simulink model "Sistema_Teste_Hugo_1"  (R2019a)
settings: Solver=ode23t  StartTime=0.0  StopTime=86400  MaxStep=6  RelTol=1e-3  EnableMultiTasking=on
InitFcn:
  | Dados_do_Sistema
undefined symbols (not defined in the file or in its folder): D1, Dados, Delta
libraries: powerlib x263, powerlib_meascontrol x79, dspsrcs4 x50
(part 5 of 5)

== system Sistema_Teste_Hugo_1/Load_8 ==
  note: Subsystem
  Add{,1..5} (6 alike) : Sum
  Ativa : Sin  Amplitude=16  Frequency=6.9e-5  Phase=-3.14  SampleTime=0
  Complex to Magnitude-Angle : ComplexToMagnitudeAngle  Output=Angle
  Constant2 : Constant  Value=-1.57079
  Controlled Current Source : powerlib/Electrical Sources/Controlled Current Source  Initialize=off  Source_Type=AC  Amplitude=0  Phase=0  Frequency=0  Measurements=None
      settings: SourceProductName=Simscape Electrical
  Controlled Current Source1 : powerlib/Electrical Sources/Controlled Current Source  Initialize=off  Source_Type=AC  Amplitude=0  Phase=0  Frequency=0  Measurements=None
      settings: SourceProductName=Simscape Electrical
  Controlled Current Source2 : powerlib/Electrical Sources/Controlled Current Source  Initialize=off  Source_Type=AC  Amplitude=0  Phase=0  Frequency=0  Measurements=None
      settings: SourceProductName=Simscape Electrical
  Demux : Demux  Outputs=3
  Demux1 : Demux  Outputs=3
  Demux2 : Demux  Outputs=3
  First-Order Filter : powerlib_meascontrol/Filters/First-Order Filter  FilterType=Lowpass  Tc=200  Ts=0  Initialize=on  Vac_Init=[0, 0, 60]  Vdc_Init=1  PlotResponse=off  FreqRange="[0,  200,  1]"
      settings: SourceProductName=Simscape Electrical
  First-Order Filter1 : powerlib_meascontrol/Filters/First-Order Filter  FilterType=Lowpass  Tc=400  Ts=0  Initialize=on  Vac_Init=[0, 0, 60]  Vdc_Init=1  PlotResponse=off  FreqRange="[0,  200,  1]"
      settings: SourceProductName=Simscape Electrical
  Gain : Gain  Gain=0.25
  Gain1 : Gain  Gain=0.25
  Gain4 : Gain  Gain=-1
  Ground2 : powerlib/Elements/Ground  LConnTagsString=a
      settings: SourceProductName=Simscape Electrical
  Magnitude-Angle to Complex{,1..5} (6 alike) : MagnitudeAngleToComplex
  Memory1 : Memory
  Memory2 : Memory
  Mux1 : Mux  Inputs=3
  Power (Phasor)2 : powerlib_meascontrol/Measurements/Power (Phasor)
      settings: SourceProductName=Simscape Electrical  SourceProductBaseCode=PS
  Product : Product
  Product1 : Product
  Random Source : dspsrcs4/Random Source  SrcType=Uniform  NormMethod=Ziggurat  CltLength=12  MinVal=0.45  MaxVal=1  MeanVal=0  VarVal=1  RepMode=Repeatable  rawSeed=1  IsInherit=off  SampMode=Discrete  SampTime=200  SampFrame=1  DataType=Single  OutComplex=Real  OutputFrames=on
  Random Source1 : dspsrcs4/Random Source  SrcType=Uniform  NormMethod=Ziggurat  CltLength=12  MinVal=0.75  MaxVal=1  MeanVal=0  VarVal=1  RepMode=Repeatable  rawSeed=1  IsInherit=off  SampMode=Discrete  SampTime=400  SampFrame=1  DataType=Single  OutComplex=Real  OutputFrames=on
  Reativa : Sin  Amplitude=5  Frequency=6.9e-5  Phase=-3.14  SampleTime=0
  Saturation : Saturate  UpperLimit=36  LowerLimit=7
  Saturation1 : Saturate  UpperLimit=10  LowerLimit=3.5
  Three-Phase Series RLC Branch2 : powerlib/Elements/Three-Phase Series RLC Branch  LConnTagsString=A|B|C  RConnTagsString=A|B|C  BranchType=RC  Resistance=0.0001  Inductance=5.46e-6  Capacitance=1e-9  Measurements=None
      settings: SourceProductName=Simscape Electrical
  Three-Phase V-I Measurement2 : powerlib/Measurements/Three-Phase V-I Measurement  VoltageMeasurement=phase-to-ground  SetLabelV=on  LabelV=VL8  Vpu=off  VpuLL=off  CurrentMeasurement=no  SetLabelI=on  LabelI=IL8  Ipu=off  Pbase=100e6  Vbase=500e3  OutputType=Complex  PhasorSimulation=on  PSBequivalent=0
      settings: SourceProductName=Simscape Electrical
  To Workspace1 : ToWorkspace  VariableName=P_Load_8_A  SampleTime=-1
  To Workspace2 : ToWorkspace  VariableName=Q_Load_8_A  SampleTime=-1
  To Workspace3 : ToWorkspace  VariableName=P_Load_8_B  SampleTime=-1
  To Workspace4 : ToWorkspace  VariableName=P_Load_8_C  SampleTime=-1
  To Workspace5 : ToWorkspace  VariableName=Q_Load_8_B  SampleTime=-1
  To Workspace6 : ToWorkspace  VariableName=Q_Load_8_C  SampleTime=-1
  i_current1 : powerlib/Measurements/Current Measurement  PhasorSimulation=on  OutputType=Complex  PSBequivalent=0
      settings: SourceProductName=Simscape Electrical
  i_current2 : powerlib/Measurements/Current Measurement  PhasorSimulation=on  OutputType=Complex  PSBequivalent=0
      settings: SourceProductName=Simscape Electrical
  i_current3 : powerlib/Measurements/Current Measurement  PhasorSimulation=on  OutputType=Complex  PSBequivalent=0
      settings: SourceProductName=Simscape Electrical
  a+ : PMIOPort  Side=Right
  b+ : PMIOPort  Port=2  Side=Right
  c+ : PMIOPort  Port=3  Side=Right
  wires:
  Ativa/1 -> Saturation/1
  Saturation/1 -> Product/2
  Random Source/1 -> First-Order Filter/1
  First-Order Filter/1 -> Product/1
  Reativa/1 -> Saturation1/1
  First-Order Filter1/1 -> Product1/1
  Random Source1/1 -> First-Order Filter1/1
  Saturation1/1 -> Product1/2
  Add/1 -> Controlled Current Source/1
  Magnitude-Angle to Complex/1 -> Add/1
  Magnitude-Angle to Complex1/1 -> Add/2
  Add1/1 -> Controlled Current Source1/1
  Magnitude-Angle to Complex2/1 -> Add1/1
  Magnitude-Angle to Complex3/1 -> Add1/2
  Add2/1 -> Controlled Current Source2/1
  Magnitude-Angle to Complex4/1 -> Add2/1
  Magnitude-Angle to Complex5/1 -> Add2/2
  Complex to Magnitude-Angle/1 -> Demux/1
  Demux/1 -> Magnitude-Angle to Complex/2, Add3/2
  Constant2/1 -> Add5/1, Add4/1, Add3/1
  Add3/1 -> Magnitude-Angle to Complex1/2
  Demux/2 -> Add4/2, Magnitude-Angle to Complex2/2
  Add4/1 -> Magnitude-Angle to Complex3/2
  Demux/3 -> Magnitude-Angle to Complex4/2, Add5/2
  Add5/1 -> Magnitude-Angle to Complex5/2
  [VL8] -> Gain4/1
  Memory1/1 -> Complex to Magnitude-Angle/1
  Product/1 -> Gain1/1, Magnitude-Angle to Complex4/1, Magnitude-Angle to Complex2/1
  Product1/1 -> Gain/1, Magnitude-Angle to Complex5/1, Magnitude-Angle to Complex3/1
  Gain1/1 -> Magnitude-Angle to Complex/1
  Gain/1 -> Magnitude-Angle to Complex1/1
  Gain4/1 -> Memory1/1
  Mux1/1 -> Power (Phasor)2/2
  Power (Phasor)2/2 -> Demux2/1
  [VL8] -> Memory2/1
  i_current1/1 -> Mux1/2
  Power (Phasor)2/1 -> Demux1/1
  Demux2/1 -> To Workspace2/1
  Demux1/2 -> To Workspace3/1
  i_current2/1 -> Mux1/3
  Demux2/3 -> To Workspace6/1
  Demux2/2 -> To Workspace5/1
  Demux1/3 -> To Workspace4/1
  Memory2/1 -> Power (Phasor)2/1
  Demux1/1 -> To Workspace1/1
  i_current3/1 -> Mux1/1
  connections:
  Three-Phase V-I Measurement2/RConn1 -- Controlled Current Source/RConn1 -- Three-Phase Series RLC Branch2/LConn1
  Three-Phase V-I Measurement2/RConn2 -- Controlled Current Source1/RConn1 -- Three-Phase Series RLC Branch2/LConn2
  Three-Phase V-I Measurement2/RConn3 -- Controlled Current Source2/RConn1 -- Three-Phase Series RLC Branch2/LConn3
  Controlled Current Source1/LConn1 -- Three-Phase Series RLC Branch2/RConn3 -- Three-Phase Series RLC Branch2/RConn1 -- Controlled Current Source/LConn1 -- Three-Phase Series RLC Branch2/RConn2 -- Ground2/LConn1 -- Controlled Current Source2/LConn1
  a+/RConn1 -- i_current3/RConn1
  Three-Phase V-I Measurement2/LConn3 -- i_current2/LConn1
  b+/RConn1 -- i_current1/RConn1
  Three-Phase V-I Measurement2/LConn1 -- i_current3/LConn1
  c+/RConn1 -- i_current2/RConn1
  Three-Phase V-I Measurement2/LConn2 -- i_current1/LConn1

== system Sistema_Teste_Hugo_1/Load_9 ==
  note: Subsystem
  Add{,1..5} (6 alike) : Sum
  Ativa : Sin  Amplitude=8  Frequency=6.9e-5  Phase=-3.14  SampleTime=0
  Complex to Magnitude-Angle : ComplexToMagnitudeAngle  Output=Angle
  Constant2 : Constant  Value=-1.57079
  Controlled Current Source : powerlib/Electrical Sources/Controlled Current Source  Initialize=off  Source_Type=AC  Amplitude=0  Phase=0  Frequency=0  Measurements=None
      settings: SourceProductName=Simscape Electrical
  Controlled Current Source1 : powerlib/Electrical Sources/Controlled Current Source  Initialize=off  Source_Type=AC  Amplitude=0  Phase=0  Frequency=0  Measurements=None
      settings: SourceProductName=Simscape Electrical
  Controlled Current Source2 : powerlib/Electrical Sources/Controlled Current Source  Initialize=off  Source_Type=AC  Amplitude=0  Phase=0  Frequency=0  Measurements=None
      settings: SourceProductName=Simscape Electrical
  Demux : Demux  Outputs=3
  Demux1 : Demux  Outputs=3
  Demux2 : Demux  Outputs=3
  First-Order Filter : powerlib_meascontrol/Filters/First-Order Filter  FilterType=Lowpass  Tc=200  Ts=0  Initialize=on  Vac_Init=[0, 0, 60]  Vdc_Init=1  PlotResponse=off  FreqRange="[0,  200,  1]"
      settings: SourceProductName=Simscape Electrical
  First-Order Filter1 : powerlib_meascontrol/Filters/First-Order Filter  FilterType=Lowpass  Tc=400  Ts=0  Initialize=on  Vac_Init=[0, 0, 60]  Vdc_Init=1  PlotResponse=off  FreqRange="[0,  200,  1]"
      settings: SourceProductName=Simscape Electrical
  Gain : Gain  Gain=0.5
  Gain1 : Gain  Gain=0.5
  Gain4 : Gain  Gain=-1
  Ground2 : powerlib/Elements/Ground  LConnTagsString=a
      settings: SourceProductName=Simscape Electrical
  Magnitude-Angle to Complex{,1..5} (6 alike) : MagnitudeAngleToComplex
  Memory1 : Memory
  Memory2 : Memory
  Mux1 : Mux  Inputs=3
  Power (Phasor)2 : powerlib_meascontrol/Measurements/Power (Phasor)
      settings: SourceProductName=Simscape Electrical  SourceProductBaseCode=PS
  Product : Product
  Product1 : Product
  Random Source : dspsrcs4/Random Source  SrcType=Uniform  NormMethod=Ziggurat  CltLength=12  MinVal=0.8  MaxVal=1  MeanVal=0  VarVal=1  RepMode=Repeatable  rawSeed=1  IsInherit=off  SampMode=Discrete  SampTime=200  SampFrame=1  DataType=Single  OutComplex=Real  OutputFrames=on
  Random Source1 : dspsrcs4/Random Source  SrcType=Uniform  NormMethod=Ziggurat  CltLength=12  MinVal=0.5  MaxVal=1  MeanVal=0  VarVal=1  RepMode=Repeatable  rawSeed=1  IsInherit=off  SampMode=Discrete  SampTime=400  SampFrame=1  DataType=Single  OutComplex=Real  OutputFrames=on
  Reativa : Sin  Amplitude=3  Frequency=6.9e-5  Phase=-3.14  SampleTime=0
  Saturation : Saturate  UpperLimit=36  LowerLimit=4
  Saturation1 : Saturate  UpperLimit=10  LowerLimit=2.5
  Three-Phase Series RLC Branch2 : powerlib/Elements/Three-Phase Series RLC Branch  LConnTagsString=A|B|C  RConnTagsString=A|B|C  BranchType=RC  Resistance=0.0001  Inductance=5.46e-6  Capacitance=1e-9  Measurements=None
      settings: SourceProductName=Simscape Electrical
  Three-Phase V-I Measurement2 : powerlib/Measurements/Three-Phase V-I Measurement  VoltageMeasurement=phase-to-ground  SetLabelV=on  LabelV=VL9  Vpu=off  VpuLL=off  CurrentMeasurement=no  SetLabelI=on  LabelI=IL9  Ipu=off  Pbase=100e6  Vbase=500e3  OutputType=Complex  PhasorSimulation=on  PSBequivalent=0
      settings: SourceProductName=Simscape Electrical
  To Workspace1 : ToWorkspace  VariableName=P_Load_9_A  SampleTime=-1
  To Workspace2 : ToWorkspace  VariableName=Q_Load_9_A  SampleTime=-1
  To Workspace3 : ToWorkspace  VariableName=P_Load_9_B  SampleTime=-1
  To Workspace4 : ToWorkspace  VariableName=P_Load_9_C  SampleTime=-1
  To Workspace5 : ToWorkspace  VariableName=Q_Load_9_B  SampleTime=-1
  To Workspace6 : ToWorkspace  VariableName=Q_Load_9_C  SampleTime=-1
  i_current1 : powerlib/Measurements/Current Measurement  PhasorSimulation=on  OutputType=Complex  PSBequivalent=0
      settings: SourceProductName=Simscape Electrical
  i_current2 : powerlib/Measurements/Current Measurement  PhasorSimulation=on  OutputType=Complex  PSBequivalent=0
      settings: SourceProductName=Simscape Electrical
  i_current3 : powerlib/Measurements/Current Measurement  PhasorSimulation=on  OutputType=Complex  PSBequivalent=0
      settings: SourceProductName=Simscape Electrical
  a+ : PMIOPort  Side=Right
  b+ : PMIOPort  Port=2  Side=Right
  c+ : PMIOPort  Port=3  Side=Right
  wires:
  Ativa/1 -> Saturation/1
  Saturation/1 -> Product/2
  Random Source/1 -> First-Order Filter/1
  First-Order Filter/1 -> Product/1
  Reativa/1 -> Saturation1/1
  First-Order Filter1/1 -> Product1/1
  Random Source1/1 -> First-Order Filter1/1
  Saturation1/1 -> Product1/2
  Add/1 -> Controlled Current Source/1
  Magnitude-Angle to Complex/1 -> Add/1
  Magnitude-Angle to Complex1/1 -> Add/2
  Add1/1 -> Controlled Current Source1/1
  Magnitude-Angle to Complex2/1 -> Add1/1
  Magnitude-Angle to Complex3/1 -> Add1/2
  Add2/1 -> Controlled Current Source2/1
  Magnitude-Angle to Complex4/1 -> Add2/1
  Magnitude-Angle to Complex5/1 -> Add2/2
  Complex to Magnitude-Angle/1 -> Demux/1
  Demux/1 -> Magnitude-Angle to Complex/2, Add3/2
  Constant2/1 -> Add5/1, Add4/1, Add3/1
  Add3/1 -> Magnitude-Angle to Complex1/2
  Demux/2 -> Add4/2, Magnitude-Angle to Complex2/2
  Add4/1 -> Magnitude-Angle to Complex3/2
  Demux/3 -> Magnitude-Angle to Complex4/2, Add5/2
  Add5/1 -> Magnitude-Angle to Complex5/2
  [VL9] -> Gain4/1
  Memory1/1 -> Complex to Magnitude-Angle/1
  Product/1 -> Magnitude-Angle to Complex/1, Magnitude-Angle to Complex4/1, Gain/1
  Product1/1 -> Magnitude-Angle to Complex1/1, Magnitude-Angle to Complex5/1, Gain1/1
  Gain/1 -> Magnitude-Angle to Complex2/1
  Gain1/1 -> Magnitude-Angle to Complex3/1
  Gain4/1 -> Memory1/1
  i_current3/1 -> Mux1/1
  Demux1/2 -> To Workspace3/1
  Mux1/1 -> Power (Phasor)2/2
  Demux2/3 -> To Workspace6/1
  Demux2/1 -> To Workspace2/1
  Demux2/2 -> To Workspace5/1
  i_current2/1 -> Mux1/3
  i_current1/1 -> Mux1/2
  Demux1/1 -> To Workspace1/1
  [VL9] -> Memory2/1
  Power (Phasor)2/1 -> Demux1/1
  Power (Phasor)2/2 -> Demux2/1
  Demux1/3 -> To Workspace4/1
  Memory2/1 -> Power (Phasor)2/1
  connections:
  Three-Phase V-I Measurement2/RConn1 -- Controlled Current Source/RConn1 -- Three-Phase Series RLC Branch2/LConn1
  Three-Phase V-I Measurement2/RConn2 -- Controlled Current Source1/RConn1 -- Three-Phase Series RLC Branch2/LConn2
  Three-Phase V-I Measurement2/RConn3 -- Controlled Current Source2/RConn1 -- Three-Phase Series RLC Branch2/LConn3
  Controlled Current Source1/LConn1 -- Three-Phase Series RLC Branch2/RConn3 -- Three-Phase Series RLC Branch2/RConn1 -- Controlled Current Source/LConn1 -- Three-Phase Series RLC Branch2/RConn2 -- Ground2/LConn1 -- Controlled Current Source2/LConn1
  Three-Phase V-I Measurement2/LConn2 -- i_current1/LConn1
  Three-Phase V-I Measurement2/LConn1 -- i_current3/LConn1
  a+/RConn1 -- i_current3/RConn1
  Three-Phase V-I Measurement2/LConn3 -- i_current2/LConn1
  b+/RConn1 -- i_current1/RConn1
  c+/RConn1 -- i_current2/RConn1

== system Sistema_Teste_Hugo_1/PV_source ==
  note: 5000 VA is the apparent power
      | of the PV inverter
  note: To change the active power values and profile,
      | you must change these four blocks.
  note: This constant block regulates the reactive current injection.
      | Here we are making the PV generate zero reactive power/current
  note: -1.5708 is the 90º phase shift of
      | reactive current
  note: Maximum power that PV can generate,
      | the MPPT should track this value
  note: power to current
      | converter
  note: Memory block to avoid
      | algebric loop due to
      | the feedback of phase
  note: Active and reactive output
      | power injected into the grid
  A_inv1 : Constant  Value=5000
  Add1 : Sum
  Add2 : Sum
  Complex to Magnitude-Angle3 : ComplexToMagnitudeAngle
  Constant1 : Constant  Value=-1.5708
  Controlled Current Source : powerlib/Electrical Sources/Controlled Current Source  Initialize=off  Source_Type=AC  Amplitude=0  Phase=0  Frequency=0  Measurements=None
      settings: SourceProductName=Simscape Electrical
  First-Order Filter : powerlib_meascontrol/Filters/First-Order Filter  FilterType=Lowpass  Tc=1000  Ts=0  Initialize=on  Vac_Init=[0, 0, 60]  Vdc_Init=1  PlotResponse=off  FreqRange="[0,  200,  1]"
      settings: SourceProductName=Simscape Electrical
  MATLAB Function : MATLAB Function  TreatAsAtomicUnit=on
  MATLAB Function1 : MATLAB Function  TreatAsAtomicUnit=on
  Magnitude-Angle to Complex : MagnitudeAngleToComplex
  Magnitude-Angle to Complex1 : MagnitudeAngleToComplex
  Math Function : Math  Operator=square  SaturateOnIntegerOverflow=on
  Math Function1 : Math  Operator=square  SaturateOnIntegerOverflow=on
  Memory1 : Memory
  Power (Phasor) : powerlib_meascontrol/Measurements/Power (Phasor)
      settings: SourceProductName=Simscape Electrical  SourceProductBaseCode=PS
  Product1 : Product
  Product2 : Product
  Product3 : Product
  Random Source : dspsrcs4/Random Source  SrcType=Uniform  NormMethod=Ziggurat  CltLength=12  MinVal=0  MaxVal=1  MeanVal=0  VarVal=1  RepMode=Not repeatable  rawSeed=1  IsInherit=off  SampMode=Discrete  SampTime=200  SampFrame=1  DataType=Single  OutComplex=Real  OutputFrames=on
  Saturation : Saturate  UpperLimit=5200  LowerLimit=0
  Scope : Scope  NumInputPorts=8
  Scope1 : Scope
  Sine Wave : Sin  Amplitude=5000  Frequency=6.9e-5  Phase=-1.57  SampleTime=0
  Sqrt : Sqrt  SaturateOnIntegerOverflow=on
  Sum1 : Sum  Inputs=|+-
  Voltage Measurement : powerlib/Measurements/Voltage Measurement  PhasorSimulation=on  OutputType=Complex  PSBequivalent=0
      settings: SourceProductName=Simscape Electrical
  i_current1 : powerlib/Measurements/Current Measurement  PhasorSimulation=on  OutputType=Complex  PSBequivalent=0
      settings: SourceProductName=Simscape Electrical
  + : PMIOPort  Side=Right
  - : PMIOPort  Port=2  Side=Right
  P_out : Outport
  Q_out : Outport  Port=2
  Pmax : Outport  Port=3
  Qmax : Outport  Port=4
  wires:
  Sine Wave/1 -> Saturation/1
  Random Source/1 -> First-Order Filter/1
  Saturation/1 -> Scope1/1, Scope/8, Scope/5, Product2/2
  First-Order Filter/1 -> Scope/7, Scope/6, Product2/1
  Add1/1 -> Controlled Current Source/1
  Voltage Measurement/1 -> Memory1/1, Power (Phasor)/1
  i_current1/1 -> Power (Phasor)/2
  Add2/1 -> Magnitude-Angle to Complex1/2
  Constant1/1 -> Add2/1
  Magnitude-Angle to Complex1/1 -> Add1/1
  Magnitude-Angle to Complex/1 -> Add1/2
  Complex to Magnitude-Angle3/2 -> Add2/2, Magnitude-Angle to Complex/2
  Complex to Magnitude-Angle3/1 -> [V_pk]
  Power (Phasor)/1 -> P_out/1
  Power (Phasor)/2 -> Q_out/1
  Memory1/1 -> Complex to Magnitude-Angle3/1
  Product2/1 -> Scope/3, Product3/2, Pmax/1
  [b] -> Product1/1
  Math Function1/1 -> Sum1/2
  Math Function/1 -> Sum1/1
  Sum1/1 -> Sqrt/1
  A_inv1/1 -> Math Function/1
  [V_pk] -> MATLAB Function/1(V_pk)
  [V_pk] -> MATLAB Function1/1(V_pk)
  Product1/1 -> Scope/2, MATLAB Function1/2(Q)
  MATLAB Function1/1(Iq) -> Magnitude-Angle to Complex1/1
  Product3/1 -> Math Function1/1, Scope/4, MATLAB Function/2(P)
  [a] -> Product3/1
  Sqrt/1 -> Scope/1, Qmax/1, Product1/2
  MATLAB Function/1(Ip) -> Magnitude-Angle to Complex/1
  connections:
  Controlled Current Source/RConn1 -- i_current1/LConn1 -- Voltage Measurement/LConn1
  Controlled Current Source/LConn1 -- Voltage Measurement/LConn2 -- -/RConn1
  i_current1/RConn1 -- +/RConn1

== system Sistema_Teste_Hugo_1/PV_source1 ==
  note: alpha_q
  note: 5000 VA is the apparent power
      | of the PV inverter
  note: To change the active power values and profile,
      | you must change these four blocks.
  note: This constant block regulates the reactive current injection.
      | Here we are making the PV generate zero reactive power/current
  note: -1.5708 is the 90º phase shift of
      | reactive current
  note: Maximum power that PV can generate,
      | the MPPT should track this value
  note: power to current
      | converter
  note: Memory block to avoid
      | algebric loop due to
      | the feedback of phase
  note: Active and reactive output
      | power injected into the grid
  note: alpha_p
  A_inv1 : Constant  Value=7000
  Add1 : Sum
  Add2 : Sum
  Complex to Magnitude-Angle3 : ComplexToMagnitudeAngle
  Constant1 : Constant  Value=-1.5708
  Controlled Current Source : powerlib/Electrical Sources/Controlled Current Source  Initialize=off  Source_Type=AC  Amplitude=0  Phase=0  Frequency=0  Measurements=None
      settings: SourceProductName=Simscape Electrical
  First-Order Filter : powerlib_meascontrol/Filters/First-Order Filter  FilterType=Lowpass  Tc=1000  Ts=0  Initialize=on  Vac_Init=[0, 0, 60]  Vdc_Init=1  PlotResponse=off  FreqRange="[0,  200,  1]"
      settings: SourceProductName=Simscape Electrical
  MATLAB Function : MATLAB Function  TreatAsAtomicUnit=on
  MATLAB Function1 : MATLAB Function  TreatAsAtomicUnit=on
  Magnitude-Angle to Complex : MagnitudeAngleToComplex
  Magnitude-Angle to Complex1 : MagnitudeAngleToComplex
  Math Function : Math  Operator=square  SaturateOnIntegerOverflow=on
  Math Function1 : Math  Operator=square  SaturateOnIntegerOverflow=on
  Memory1 : Memory
  Power (Phasor) : powerlib_meascontrol/Measurements/Power (Phasor)
      settings: SourceProductName=Simscape Electrical  SourceProductBaseCode=PS
  Product1 : Product
  Product2 : Product
  Product3 : Product
  Random Source : dspsrcs4/Random Source  SrcType=Uniform  NormMethod=Ziggurat  CltLength=12  MinVal=0  MaxVal=1  MeanVal=0  VarVal=1  RepMode=Not repeatable  rawSeed=1  IsInherit=off  SampMode=Discrete  SampTime=200  SampFrame=1  DataType=Single  OutComplex=Real  OutputFrames=on
  Saturation : Saturate  UpperLimit=7200  LowerLimit=0
  Sine Wave : Sin  Amplitude=7000  Frequency=6.9e-5  Phase=-1.57  SampleTime=0
  Sqrt : Sqrt  SaturateOnIntegerOverflow=on
  Sum1 : Sum  Inputs=|+-
  Voltage Measurement : powerlib/Measurements/Voltage Measurement  PhasorSimulation=on  OutputType=Complex  PSBequivalent=0
      settings: SourceProductName=Simscape Electrical
  i_current1 : powerlib/Measurements/Current Measurement  PhasorSimulation=on  OutputType=Complex  PSBequivalent=0
      settings: SourceProductName=Simscape Electrical
  + : PMIOPort  Side=Right
  - : PMIOPort  Port=2  Side=Right
  P_out : Outport
  Q_out : Outport  Port=2
  Pmax : Outport  Port=3
  Qmax : Outport  Port=4
  wires:
  Sine Wave/1 -> Saturation/1
  Random Source/1 -> First-Order Filter/1
  Saturation/1 -> Product2/2
  First-Order Filter/1 -> Product2/1
  Add1/1 -> Controlled Current Source/1
  Voltage Measurement/1 -> Memory1/1, Power (Phasor)/1
  i_current1/1 -> Power (Phasor)/2
  Add2/1 -> Magnitude-Angle to Complex1/2
  Constant1/1 -> Add2/1
  Magnitude-Angle to Complex1/1 -> Add1/1
  Magnitude-Angle to Complex/1 -> Add1/2
  Complex to Magnitude-Angle3/2 -> Add2/2, Magnitude-Angle to Complex/2
  Complex to Magnitude-Angle3/1 -> [V_pk]
  Power (Phasor)/1 -> P_out/1
  Power (Phasor)/2 -> Q_out/1
  Memory1/1 -> Complex to Magnitude-Angle3/1
  Product2/1 -> Product3/2, Pmax/1
  [b] -> Product1/1
  Math Function1/1 -> Sum1/2
  Math Function/1 -> Sum1/1
  Sum1/1 -> Sqrt/1
  A_inv1/1 -> Math Function/1
  MATLAB Function/1(Ip) -> Magnitude-Angle to Complex/1
  Sqrt/1 -> Qmax/1, Product1/2
  [V_pk] -> MATLAB Function/1(V_pk)
  [V_pk] -> MATLAB Function1/1(V_pk)
  Product1/1 -> MATLAB Function1/2(Q)
  MATLAB Function1/1(Iq) -> Magnitude-Angle to Complex1/1
  Product3/1 -> Math Function1/1, MATLAB Function/2(P)
  [a] -> Product3/1
  connections:
  Controlled Current Source/RConn1 -- i_current1/LConn1 -- Voltage Measurement/LConn1
  Controlled Current Source/LConn1 -- Voltage Measurement/LConn2 -- -/RConn1
  i_current1/RConn1 -- +/RConn1

== system Sistema_Teste_Hugo_1/PV_source2 ==
  note: alpha_q
  note: 5000 VA is the apparent power
      | of the PV inverter
  note: To change the active power values and profile,
      | you must change these four blocks.
  note: This constant block regulates the reactive current injection.
      | Here we are making the PV generate zero reactive power/current
  note: -1.5708 is the 90º phase shift of
      | reactive current
  note: Maximum power that PV can generate,
      | the MPPT should track this value
  note: power to current
      | converter
  note: Memory block to avoid
      | algebric loop due to
      | the feedback of phase
  note: Active and reactive output
      | power injected into the grid
  note: alpha_p
  A_inv1 : Constant  Value=5000
  Add1 : Sum
  Add2 : Sum
  Complex to Magnitude-Angle3 : ComplexToMagnitudeAngle
  Constant1 : Constant  Value=-1.5708
  Controlled Current Source : powerlib/Electrical Sources/Controlled Current Source  Initialize=off  Source_Type=AC  Amplitude=0  Phase=0  Frequency=0  Measurements=None
      settings: SourceProductName=Simscape Electrical
  First-Order Filter : powerlib_meascontrol/Filters/First-Order Filter  FilterType=Lowpass  Tc=1000  Ts=0  Initialize=on  Vac_Init=[0, 0, 60]  Vdc_Init=1  PlotResponse=off  FreqRange="[0,  200,  1]"
      settings: SourceProductName=Simscape Electrical
  MATLAB Function : MATLAB Function  TreatAsAtomicUnit=on
  MATLAB Function1 : MATLAB Function  TreatAsAtomicUnit=on
  Magnitude-Angle to Complex : MagnitudeAngleToComplex
  Magnitude-Angle to Complex1 : MagnitudeAngleToComplex
  Math Function : Math  Operator=square  SaturateOnIntegerOverflow=on
  Math Function1 : Math  Operator=square  SaturateOnIntegerOverflow=on
  Memory1 : Memory
  Power (Phasor) : powerlib_meascontrol/Measurements/Power (Phasor)
      settings: SourceProductName=Simscape Electrical  SourceProductBaseCode=PS
  Product1 : Product
  Product2 : Product
  Product3 : Product
  Random Source : dspsrcs4/Random Source  SrcType=Uniform  NormMethod=Ziggurat  CltLength=12  MinVal=0  MaxVal=1  MeanVal=0  VarVal=1  RepMode=Not repeatable  rawSeed=1  IsInherit=off  SampMode=Discrete  SampTime=200  SampFrame=1  DataType=Single  OutComplex=Real  OutputFrames=on
  Saturation : Saturate  UpperLimit=7200  LowerLimit=0
  Sine Wave : Sin  Amplitude=5000  Frequency=6.9e-5  Phase=-1.57  SampleTime=0
  Sqrt : Sqrt  SaturateOnIntegerOverflow=on
  Sum1 : Sum  Inputs=|+-
  Voltage Measurement : powerlib/Measurements/Voltage Measurement  PhasorSimulation=on  OutputType=Complex  PSBequivalent=0
      settings: SourceProductName=Simscape Electrical
  i_current1 : powerlib/Measurements/Current Measurement  PhasorSimulation=on  OutputType=Complex  PSBequivalent=0
      settings: SourceProductName=Simscape Electrical
  + : PMIOPort  Side=Right
  - : PMIOPort  Port=2  Side=Right
  P_out : Outport
  Q_out : Outport  Port=2
  Pmax : Outport  Port=3
  Qmax : Outport  Port=4
  wires:
  Sine Wave/1 -> Saturation/1
  Random Source/1 -> First-Order Filter/1
  Saturation/1 -> Product2/2
  First-Order Filter/1 -> Product2/1
  Add1/1 -> Controlled Current Source/1
  Voltage Measurement/1 -> Memory1/1, Power (Phasor)/1
  i_current1/1 -> Power (Phasor)/2
  Add2/1 -> Magnitude-Angle to Complex1/2
  Constant1/1 -> Add2/1
  Magnitude-Angle to Complex1/1 -> Add1/1
  Magnitude-Angle to Complex/1 -> Add1/2
  Complex to Magnitude-Angle3/2 -> Add2/2, Magnitude-Angle to Complex/2
  Complex to Magnitude-Angle3/1 -> [V_pk]
  Power (Phasor)/1 -> P_out/1
  Power (Phasor)/2 -> Q_out/1
  Memory1/1 -> Complex to Magnitude-Angle3/1
  Product2/1 -> Product3/2, Pmax/1
  [b] -> Product1/1
  Math Function1/1 -> Sum1/2
  Math Function/1 -> Sum1/1
  Sum1/1 -> Sqrt/1
  A_inv1/1 -> Math Function/1
  MATLAB Function/1(Ip) -> Magnitude-Angle to Complex/1
  Sqrt/1 -> Qmax/1, Product1/2
  [V_pk] -> MATLAB Function/1(V_pk)
  [V_pk] -> MATLAB Function1/1(V_pk)
  Product1/1 -> MATLAB Function1/2(Q)
  MATLAB Function1/1(Iq) -> Magnitude-Angle to Complex1/1
  Product3/1 -> Math Function1/1, MATLAB Function/2(P)
  [a] -> Product3/1
  connections:
  Controlled Current Source/RConn1 -- i_current1/LConn1 -- Voltage Measurement/LConn1
  Controlled Current Source/LConn1 -- Voltage Measurement/LConn2 -- -/RConn1
  i_current1/RConn1 -- +/RConn1

== system Sistema_Teste_Hugo_1/PV_source3 ==
  note: alpha_q
  note: 5000 VA is the apparent power
      | of the PV inverter
  note: To change the active power values and profile,
      | you must change these four blocks.
  note: This constant block regulates the reactive current injection.
      | Here we are making the PV generate zero reactive power/current
  note: -1.5708 is the 90º phase shift of
      | reactive current
  note: Maximum power that PV can generate,
      | the MPPT should track this value
  note: power to current
      | converter
  note: Memory block to avoid
      | algebric loop due to
      | the feedback of phase
  note: Active and reactive output
      | power injected into the grid
  note: alpha_p
  A_inv1 : Constant  Value=10000
  Add1 : Sum
  Add2 : Sum
  Complex to Magnitude-Angle3 : ComplexToMagnitudeAngle
  Constant1 : Constant  Value=-1.5708
  Controlled Current Source : powerlib/Electrical Sources/Controlled Current Source  Initialize=off  Source_Type=AC  Amplitude=0  Phase=0  Frequency=0  Measurements=None
      settings: SourceProductName=Simscape Electrical
  First-Order Filter : powerlib_meascontrol/Filters/First-Order Filter  FilterType=Lowpass  Tc=1000  Ts=0  Initialize=on  Vac_Init=[0, 0, 60]  Vdc_Init=1  PlotResponse=off  FreqRange="[0,  200,  1]"
      settings: SourceProductName=Simscape Electrical
  MATLAB Function : MATLAB Function  TreatAsAtomicUnit=on
  MATLAB Function1 : MATLAB Function  TreatAsAtomicUnit=on
  Magnitude-Angle to Complex : MagnitudeAngleToComplex
  Magnitude-Angle to Complex1 : MagnitudeAngleToComplex
  Math Function : Math  Operator=square  SaturateOnIntegerOverflow=on
  Math Function1 : Math  Operator=square  SaturateOnIntegerOverflow=on
  Memory1 : Memory
  Power (Phasor) : powerlib_meascontrol/Measurements/Power (Phasor)
      settings: SourceProductName=Simscape Electrical  SourceProductBaseCode=PS
  Product1 : Product
  Product2 : Product
  Product3 : Product
  Random Source : dspsrcs4/Random Source  SrcType=Uniform  NormMethod=Ziggurat  CltLength=12  MinVal=0  MaxVal=1  MeanVal=0  VarVal=1  RepMode=Not repeatable  rawSeed=1  IsInherit=off  SampMode=Discrete  SampTime=200  SampFrame=1  DataType=Single  OutComplex=Real  OutputFrames=on
  Saturation : Saturate  UpperLimit=10200  LowerLimit=0
  Sine Wave : Sin  Amplitude=10000  Frequency=6.9e-5  Phase=-1.57  SampleTime=0
  Sqrt : Sqrt  SaturateOnIntegerOverflow=on
  Sum1 : Sum  Inputs=|+-
  Voltage Measurement : powerlib/Measurements/Voltage Measurement  PhasorSimulation=on  OutputType=Complex  PSBequivalent=0
      settings: SourceProductName=Simscape Electrical
  i_current1 : powerlib/Measurements/Current Measurement  PhasorSimulation=on  OutputType=Complex  PSBequivalent=0
      settings: SourceProductName=Simscape Electrical
  + : PMIOPort  Side=Right
  - : PMIOPort  Port=2  Side=Right
  P_out : Outport
  Q_out : Outport  Port=2
  Pmax : Outport  Port=3
  Qmax : Outport  Port=4
  wires:
  Sine Wave/1 -> Saturation/1
  Random Source/1 -> First-Order Filter/1
  Saturation/1 -> Product2/2
  First-Order Filter/1 -> Product2/1
  Add1/1 -> Controlled Current Source/1
  Voltage Measurement/1 -> Memory1/1, Power (Phasor)/1
  i_current1/1 -> Power (Phasor)/2
  Add2/1 -> Magnitude-Angle to Complex1/2
  Constant1/1 -> Add2/1
  Magnitude-Angle to Complex1/1 -> Add1/1
  Magnitude-Angle to Complex/1 -> Add1/2
  Complex to Magnitude-Angle3/2 -> Add2/2, Magnitude-Angle to Complex/2
  Complex to Magnitude-Angle3/1 -> [V_pk]
  Power (Phasor)/1 -> P_out/1
  Power (Phasor)/2 -> Q_out/1
  Memory1/1 -> Complex to Magnitude-Angle3/1
  Product2/1 -> Product3/2, Pmax/1
  [b] -> Product1/1
  Math Function1/1 -> Sum1/2
  Math Function/1 -> Sum1/1
  Sum1/1 -> Sqrt/1
  A_inv1/1 -> Math Function/1
  MATLAB Function/1(Ip) -> Magnitude-Angle to Complex/1
  Sqrt/1 -> Qmax/1, Product1/2
  [V_pk] -> MATLAB Function/1(V_pk)
  [V_pk] -> MATLAB Function1/1(V_pk)
  Product1/1 -> MATLAB Function1/2(Q)
  MATLAB Function1/1(Iq) -> Magnitude-Angle to Complex1/1
  Product3/1 -> Math Function1/1, MATLAB Function/2(P)
  [a] -> Product3/1
  connections:
  Controlled Current Source/RConn1 -- i_current1/LConn1 -- Voltage Measurement/LConn1
  Controlled Current Source/LConn1 -- Voltage Measurement/LConn2 -- -/RConn1
  i_current1/RConn1 -- +/RConn1

== system Sistema_Teste_Hugo_1/PV_source4 ==
  note: alpha_q
  note: 5000 VA is the apparent power
      | of the PV inverter
  note: To change the active power values and profile,
      | you must change these four blocks.
  note: This constant block regulates the reactive current injection.
      | Here we are making the PV generate zero reactive power/current
  note: -1.5708 is the 90º phase shift of
      | reactive current
  note: Maximum power that PV can generate,
      | the MPPT should track this value
  note: power to current
      | converter
  note: Memory block to avoid
      | algebric loop due to
      | the feedback of phase
  note: Active and reactive output
      | power injected into the grid
  note: alpha_p
  A_inv1 : Constant  Value=9000
  Add1 : Sum
  Add2 : Sum
  Complex to Magnitude-Angle3 : ComplexToMagnitudeAngle
  Constant1 : Constant  Value=-1.5708
  Controlled Current Source : powerlib/Electrical Sources/Controlled Current Source  Initialize=off  Source_Type=AC  Amplitude=0  Phase=0  Frequency=0  Measurements=None
      settings: SourceProductName=Simscape Electrical
  First-Order Filter : powerlib_meascontrol/Filters/First-Order Filter  FilterType=Lowpass  Tc=1000  Ts=0  Initialize=on  Vac_Init=[0, 0, 60]  Vdc_Init=1  PlotResponse=off  FreqRange="[0,  200,  1]"
      settings: SourceProductName=Simscape Electrical
  MATLAB Function : MATLAB Function  TreatAsAtomicUnit=on
  MATLAB Function1 : MATLAB Function  TreatAsAtomicUnit=on
  Magnitude-Angle to Complex : MagnitudeAngleToComplex
  Magnitude-Angle to Complex1 : MagnitudeAngleToComplex
  Math Function : Math  Operator=square  SaturateOnIntegerOverflow=on
  Math Function1 : Math  Operator=square  SaturateOnIntegerOverflow=on
  Memory1 : Memory
  Power (Phasor) : powerlib_meascontrol/Measurements/Power (Phasor)
      settings: SourceProductName=Simscape Electrical  SourceProductBaseCode=PS
  Product1 : Product
  Product2 : Product
  Product3 : Product
  Random Source : dspsrcs4/Random Source  SrcType=Uniform  NormMethod=Ziggurat  CltLength=12  MinVal=0  MaxVal=1  MeanVal=0  VarVal=1  RepMode=Not repeatable  rawSeed=1  IsInherit=off  SampMode=Discrete  SampTime=200  SampFrame=1  DataType=Single  OutComplex=Real  OutputFrames=on
  Saturation : Saturate  UpperLimit=10200  LowerLimit=0
  Sine Wave : Sin  Amplitude=9000  Frequency=6.9e-5  Phase=-1.57  SampleTime=0
  Sqrt : Sqrt  SaturateOnIntegerOverflow=on
  Sum1 : Sum  Inputs=|+-
  Voltage Measurement : powerlib/Measurements/Voltage Measurement  PhasorSimulation=on  OutputType=Complex  PSBequivalent=0
      settings: SourceProductName=Simscape Electrical
  i_current1 : powerlib/Measurements/Current Measurement  PhasorSimulation=on  OutputType=Complex  PSBequivalent=0
      settings: SourceProductName=Simscape Electrical
  + : PMIOPort  Side=Right
  - : PMIOPort  Port=2  Side=Right
  P_out : Outport
  Q_out : Outport  Port=2
  Pmax : Outport  Port=3
  Qmax : Outport  Port=4
  wires:
  Sine Wave/1 -> Saturation/1
  Random Source/1 -> First-Order Filter/1
  Saturation/1 -> Product2/2
  First-Order Filter/1 -> Product2/1
  Add1/1 -> Controlled Current Source/1
  Voltage Measurement/1 -> Memory1/1, Power (Phasor)/1
  i_current1/1 -> Power (Phasor)/2
  Add2/1 -> Magnitude-Angle to Complex1/2
  Constant1/1 -> Add2/1
  Magnitude-Angle to Complex1/1 -> Add1/1
  Magnitude-Angle to Complex/1 -> Add1/2
  Complex to Magnitude-Angle3/2 -> Add2/2, Magnitude-Angle to Complex/2
  Complex to Magnitude-Angle3/1 -> [V_pk]
  Power (Phasor)/1 -> P_out/1
  Power (Phasor)/2 -> Q_out/1
  Memory1/1 -> Complex to Magnitude-Angle3/1
  Product2/1 -> Product3/2, Pmax/1
  [b] -> Product1/1
  Math Function1/1 -> Sum1/2
  Math Function/1 -> Sum1/1
  Sum1/1 -> Sqrt/1
  A_inv1/1 -> Math Function/1
  MATLAB Function/1(Ip) -> Magnitude-Angle to Complex/1
  Sqrt/1 -> Qmax/1, Product1/2
  [V_pk] -> MATLAB Function/1(V_pk)
  [V_pk] -> MATLAB Function1/1(V_pk)
  Product1/1 -> MATLAB Function1/2(Q)
  MATLAB Function1/1(Iq) -> Magnitude-Angle to Complex1/1
  Product3/1 -> Math Function1/1, MATLAB Function/2(P)
  [a] -> Product3/1
  connections:
  Controlled Current Source/RConn1 -- i_current1/LConn1 -- Voltage Measurement/LConn1
  Controlled Current Source/LConn1 -- Voltage Measurement/LConn2 -- -/RConn1
  i_current1/RConn1 -- +/RConn1

== system Sistema_Teste_Hugo_1/PV_source5 ==
  note: alpha_q
  note: 5000 VA is the apparent power
      | of the PV inverter
  note: To change the active power values and profile,
      | you must change these four blocks.
  note: This constant block regulates the reactive current injection.
      | Here we are making the PV generate zero reactive power/current
  note: -1.5708 is the 90º phase shift of
      | reactive current
  note: Maximum power that PV can generate,
      | the MPPT should track this value
  note: power to current
      | converter
  note: Memory block to avoid
      | algebric loop due to
      | the feedback of phase
  note: Active and reactive output
      | power injected into the grid
  note: alpha_p
  A_inv1 : Constant  Value=9000
  Add1 : Sum
  Add2 : Sum
  Complex to Magnitude-Angle3 : ComplexToMagnitudeAngle
  Constant1 : Constant  Value=-1.5708
  Controlled Current Source : powerlib/Electrical Sources/Controlled Current Source  Initialize=off  Source_Type=AC  Amplitude=0  Phase=0  Frequency=0  Measurements=None
      settings: SourceProductName=Simscape Electrical
  First-Order Filter : powerlib_meascontrol/Filters/First-Order Filter  FilterType=Lowpass  Tc=1000  Ts=0  Initialize=on  Vac_Init=[0, 0, 60]  Vdc_Init=1  PlotResponse=off  FreqRange="[0,  200,  1]"
      settings: SourceProductName=Simscape Electrical
  MATLAB Function : MATLAB Function  TreatAsAtomicUnit=on
  MATLAB Function1 : MATLAB Function  TreatAsAtomicUnit=on
  Magnitude-Angle to Complex : MagnitudeAngleToComplex
  Magnitude-Angle to Complex1 : MagnitudeAngleToComplex
  Math Function : Math  Operator=square  SaturateOnIntegerOverflow=on
  Math Function1 : Math  Operator=square  SaturateOnIntegerOverflow=on
  Memory1 : Memory
  Power (Phasor) : powerlib_meascontrol/Measurements/Power (Phasor)
      settings: SourceProductName=Simscape Electrical  SourceProductBaseCode=PS
  Product1 : Product
  Product2 : Product
  Product3 : Product
  Random Source : dspsrcs4/Random Source  SrcType=Uniform  NormMethod=Ziggurat  CltLength=12  MinVal=0  MaxVal=1  MeanVal=0  VarVal=1  RepMode=Not repeatable  rawSeed=1  IsInherit=off  SampMode=Discrete  SampTime=200  SampFrame=1  DataType=Single  OutComplex=Real  OutputFrames=on
  Saturation : Saturate  UpperLimit=10200  LowerLimit=0
  Sine Wave : Sin  Amplitude=9000  Frequency=6.9e-5  Phase=-1.57  SampleTime=0
  Sqrt : Sqrt  SaturateOnIntegerOverflow=on
  Sum1 : Sum  Inputs=|+-
  Voltage Measurement : powerlib/Measurements/Voltage Measurement  PhasorSimulation=on  OutputType=Complex  PSBequivalent=0
      settings: SourceProductName=Simscape Electrical
  i_current1 : powerlib/Measurements/Current Measurement  PhasorSimulation=on  OutputType=Complex  PSBequivalent=0
      settings: SourceProductName=Simscape Electrical
  + : PMIOPort  Side=Right
  - : PMIOPort  Port=2  Side=Right
  P_out : Outport
  Q_out : Outport  Port=2
  Pmax : Outport  Port=3
  Qmax : Outport  Port=4
  wires:
  Sine Wave/1 -> Saturation/1
  Random Source/1 -> First-Order Filter/1
  Saturation/1 -> Product2/2
  First-Order Filter/1 -> Product2/1
  Add1/1 -> Controlled Current Source/1
  Voltage Measurement/1 -> Memory1/1, Power (Phasor)/1
  i_current1/1 -> Power (Phasor)/2
  Add2/1 -> Magnitude-Angle to Complex1/2
  Constant1/1 -> Add2/1
  Magnitude-Angle to Complex1/1 -> Add1/1
  Magnitude-Angle to Complex/1 -> Add1/2
  Complex to Magnitude-Angle3/2 -> Add2/2, Magnitude-Angle to Complex/2
  Complex to Magnitude-Angle3/1 -> [V_pk]
  Power (Phasor)/1 -> P_out/1
  Power (Phasor)/2 -> Q_out/1
  Memory1/1 -> Complex to Magnitude-Angle3/1
  Product2/1 -> Product3/2, Pmax/1
  [b] -> Product1/1
  Math Function1/1 -> Sum1/2
  Math Function/1 -> Sum1/1
  Sum1/1 -> Sqrt/1
  A_inv1/1 -> Math Function/1
  MATLAB Function/1(Ip) -> Magnitude-Angle to Complex/1
  Sqrt/1 -> Qmax/1, Product1/2
  [V_pk] -> MATLAB Function/1(V_pk)
  [V_pk] -> MATLAB Function1/1(V_pk)
  Product1/1 -> MATLAB Function1/2(Q)
  MATLAB Function1/1(Iq) -> Magnitude-Angle to Complex1/1
  Product3/1 -> Math Function1/1, MATLAB Function/2(P)
  [a] -> Product3/1
  connections:
  Controlled Current Source/RConn1 -- i_current1/LConn1 -- Voltage Measurement/LConn1
  Controlled Current Source/LConn1 -- Voltage Measurement/LConn2 -- -/RConn1
  i_current1/RConn1 -- +/RConn1

== matlab function Sistema_Teste_Hugo_1/PV_source/MATLAB Function1 ==
  data: Iq output; V_pk input; Q input
function Iq  = fcn(V_pk, Q)
%#codegen
Iq=0;
if(V_pk > 20)
Iq = 2*Q/V_pk;
end

== matlab function Sistema_Teste_Hugo_1/PV_source/MATLAB Function ==
  data: Ip output; V_pk input; P input
function Ip  = fcn(V_pk, P)
%#codegen
Ip=0;
if(V_pk > 20)
Ip = 2*P/V_pk;
end

== matlab function Sistema_Teste_Hugo_1/PV_source1/MATLAB Function ==
  data: Ip output; V_pk input; P input
function Ip  = fcn(V_pk, P)
%#codegen
Ip=0;
if(V_pk > 20)
Ip = 2*P/V_pk;
end

== matlab function Sistema_Teste_Hugo_1/PV_source1/MATLAB Function1 ==
  data: Iq output; V_pk input; Q input
function Iq  = fcn(V_pk, Q)
%#codegen
Iq=0;
if(V_pk > 20)
Iq = 2*Q/V_pk;
end

== matlab function Sistema_Teste_Hugo_1/PV_source2/MATLAB Function ==
  data: Ip output; V_pk input; P input
function Ip  = fcn(V_pk, P)
%#codegen
Ip=0;
if(V_pk > 20)
Ip = 2*P/V_pk;
end

== matlab function Sistema_Teste_Hugo_1/PV_source2/MATLAB Function1 ==
  data: Iq output; V_pk input; Q input
function Iq  = fcn(V_pk, Q)
%#codegen
Iq=0;
if(V_pk > 20)
Iq = 2*Q/V_pk;
end

== matlab function Sistema_Teste_Hugo_1/PV_source3/MATLAB Function ==
  data: Ip output; V_pk input; P input
function Ip  = fcn(V_pk, P)
%#codegen
Ip=0;
if(V_pk > 20)
Ip = 2*P/V_pk;
end

== matlab function Sistema_Teste_Hugo_1/PV_source3/MATLAB Function1 ==
  data: Iq output; V_pk input; Q input
function Iq  = fcn(V_pk, Q)
%#codegen
Iq=0;
if(V_pk > 20)
Iq = 2*Q/V_pk;
end

== matlab function Sistema_Teste_Hugo_1/PV_source4/MATLAB Function ==
  data: Ip output; V_pk input; P input
function Ip  = fcn(V_pk, P)
%#codegen
Ip=0;
if(V_pk > 20)
Ip = 2*P/V_pk;
end

== matlab function Sistema_Teste_Hugo_1/PV_source4/MATLAB Function1 ==
  data: Iq output; V_pk input; Q input
function Iq  = fcn(V_pk, Q)
%#codegen
Iq=0;
if(V_pk > 20)
Iq = 2*Q/V_pk;
end

== matlab function Sistema_Teste_Hugo_1/PV_source5/MATLAB Function ==
  data: Ip output; V_pk input; P input
function Ip  = fcn(V_pk, P)
%#codegen
Ip=0;
if(V_pk > 20)
Ip = 2*P/V_pk;
end

== matlab function Sistema_Teste_Hugo_1/PV_source5/MATLAB Function1 ==
  data: Iq output; V_pk input; Q input
function Iq  = fcn(V_pk, Q)
%#codegen
Iq=0;
if(V_pk > 20)
Iq = 2*Q/V_pk;
end

== matlab function Sistema_Teste_Hugo_1/MATLAB Function ==
  data: PG input; a output; b output; PL output; QL output; QG input; PGD input; QGD input; Pmax input; Qmax input; P0 input; Q0 input; Test1 output; Test2 output
function [a,b,PL,QL,Test1,Test2] = fcn(PG,QG,PGD,QGD,Pmax,Qmax,P0,Q0)

% a=1;
% b=0;
PL = PG+PGD;
QL = QG+QGD;

a = (PL-P0)/Pmax;
if(a>=1)
    a=1;
else if(a<=0)
        a=0;
    end
end
    
b = (QL-Q0)/Qmax;
if(b>=1)
    b=1;
else if(b<=-1)
        b=-1;
    end
end

Test1 = PL-P0;
Test2 = Pmax;

== matlab function Sistema_Teste_Hugo_1/MATLAB Function3 ==
  data: Vmax input; DesvioTensaoPCC output; Va_PCC input; Vb_PCC input; Vc_PCC input; Vmin input
function DesvioTensaoPCC  = fcn(Vmax,Va_PCC,Vb_PCC,Vc_PCC,Vmin)
%#codegen

DesvioTensaoPCC = (((Vmax - Vmin)*3)/(Va_PCC + Vb_PCC + Vc_PCC))*100;
